simulink model "torques"  (R2015a)
settings: Solver=ode45  StartTime=0.0  StopTime=10.0  RelTol=1e-3
undefined symbols (not defined in the file): Jw_fl, Jw_fr, Jw_rl, Jw_rr
settings Model: Creator=BML  LastModifiedBy=BML

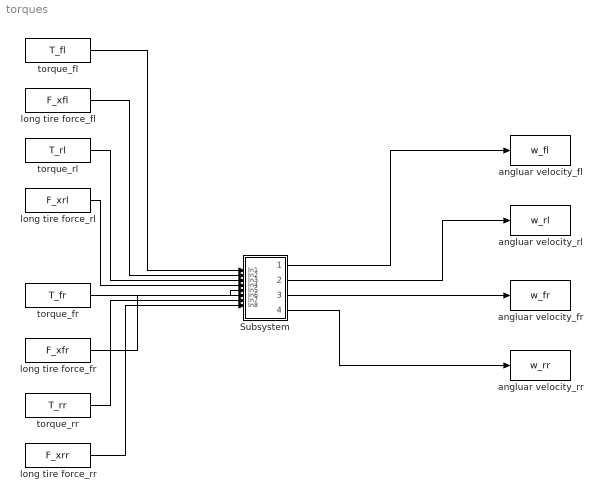
== system torques ==
  Subsystem : Subsystem
  angluar velocity_fl : ToWorkspace  VariableName=w_fl  SaveFormat=Timeseries  SampleTime=-1
  angluar velocity_fr : ToWorkspace  VariableName=w_fr  SaveFormat=Timeseries  SampleTime=-1
  angluar velocity_rl : ToWorkspace  VariableName=w_rl  SaveFormat=Timeseries  SampleTime=-1
  angluar velocity_rr : ToWorkspace  VariableName=w_rr  SaveFormat=Timeseries  SampleTime=-1
  long tire force_fl : FromWorkspace  VariableName=F_xfl  SampleTime=0
  long tire force_fr : FromWorkspace  VariableName=F_xfr  SampleTime=0
  long tire force_rl : FromWorkspace  VariableName=F_xrl  SampleTime=0
  long tire force_rr : FromWorkspace  VariableName=F_xrr  SampleTime=0
  torque_fl : FromWorkspace  VariableName=T_fl  SampleTime=0
  torque_fr : FromWorkspace  VariableName=T_fr  SampleTime=0
  torque_rl : FromWorkspace  VariableName=T_rl  SampleTime=0
  torque_rr : FromWorkspace  VariableName=T_rr  SampleTime=0
  wires:
  torque_fl/1 -> Subsystem/1(In1)
  long tire force_fl/1 -> Subsystem/2(In2)
  torque_rl/1 -> Subsystem/3(In3)
  long tire force_rl/1 -> Subsystem/4(In4)
  torque_fr/1 -> Subsystem/5(In5)
  long tire force_fr/1 -> Subsystem/6(In6)
  torque_rr/1 -> Subsystem/7(In7)
  long tire force_rr/1 -> Subsystem/8(In8)
  Subsystem/1(Out1) -> angluar velocity_fl/1
  Subsystem/2(Out2) -> angluar velocity_rl/1
  Subsystem/3(Out3) -> angluar velocity_fr/1
  Subsystem/4(Out4) -> angluar velocity_rr/1

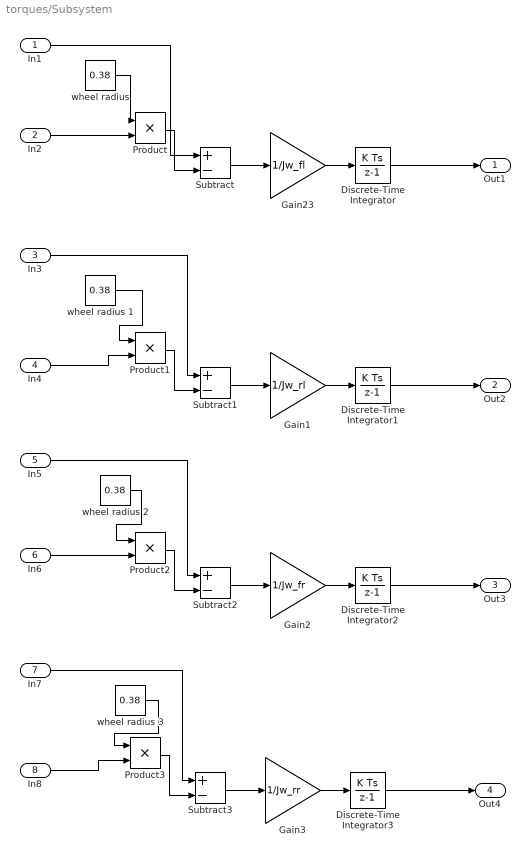
== system torques/Subsystem ==
  In1 : Inport
  In2 : Inport  Port=2
  In3 : Inport  Port=3
  In4 : Inport  Port=4
  In5 : Inport  Port=5
  In6 : Inport  Port=6
  In7 : Inport  Port=7
  In8 : Inport  Port=8
  Discrete-Time Integrator{,1..3} (4 alike) : DiscreteIntegrator  InitialConditionSetting=State (most efficient)
  Gain1 : Gain  Gain=1/Jw_rl
  Gain2 : Gain  Gain=1/Jw_fr
  Gain23 : Gain  Gain=1/Jw_fl
  Gain3 : Gain  Gain=1/Jw_rr
  Product{,1..3} (4 alike) : Product
  Subtract{,1..3} (4 alike) : Sum  Inputs=+-
  wheel radius {,1..3} (4 alike) : Constant  Value=0.38
  Out1 : Outport
  Out2 : Outport  Port=2
  Out3 : Outport  Port=3
  Out4 : Outport  Port=4
  wires:
  Gain23/1 -> Discrete-Time Integrator/1
  Discrete-Time Integrator/1 -> Out1/1
  In2/1 -> Product/2
  Product/1 -> Subtract/2
  wheel radius 1/1 -> Product1/1
  In3/1 -> Subtract1/1
  In1/1 -> Subtract/1
  Subtract/1 -> Gain23/1
  In4/1 -> Product1/2
  "wheel radius "/1 -> Product/1
  Subtract2/1 -> Gain2/1
  wheel radius 2/1 -> Product2/1
  Product1/1 -> Subtract1/2
  In8/1 -> Product3/2
  In7/1 -> Subtract3/1
  Gain3/1 -> Discrete-Time Integrator3/1
  Subtract1/1 -> Gain1/1
  Gain1/1 -> Discrete-Time Integrator1/1
  Gain2/1 -> Discrete-Time Integrator2/1
  Subtract3/1 -> Gain3/1
  Discrete-Time Integrator3/1 -> Out4/1
  wheel radius 3/1 -> Product3/1
  In6/1 -> Product2/2
  Product3/1 -> Subtract3/2
  In5/1 -> Subtract2/1
  Product2/1 -> Subtract2/2
  Discrete-Time Integrator1/1 -> Out2/1
  Discrete-Time Integrator2/1 -> Out3/1
